simulink model "LQ_Controller"  (R2022b)
settings: Solver=ode45  StartTime=0.0  StopTime=15.0  MaxStep=0.001  RelTol=1e-5
undefined symbols (not defined in the file or in its folder): A, B, C, D, Klqi, Klqp
settings Model: Creator=emanuela  LastModifiedBy=emanuela
settings DataIOCC: SaveOutput=off  SignalLogging=off  DSMLogging=off  SaveTime=off  ReturnWorkspaceOutputs=off

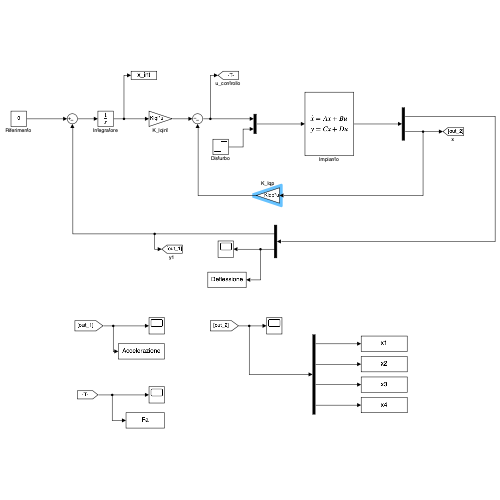
[thumbnail: Simulink's stored preview of the top-level diagram]
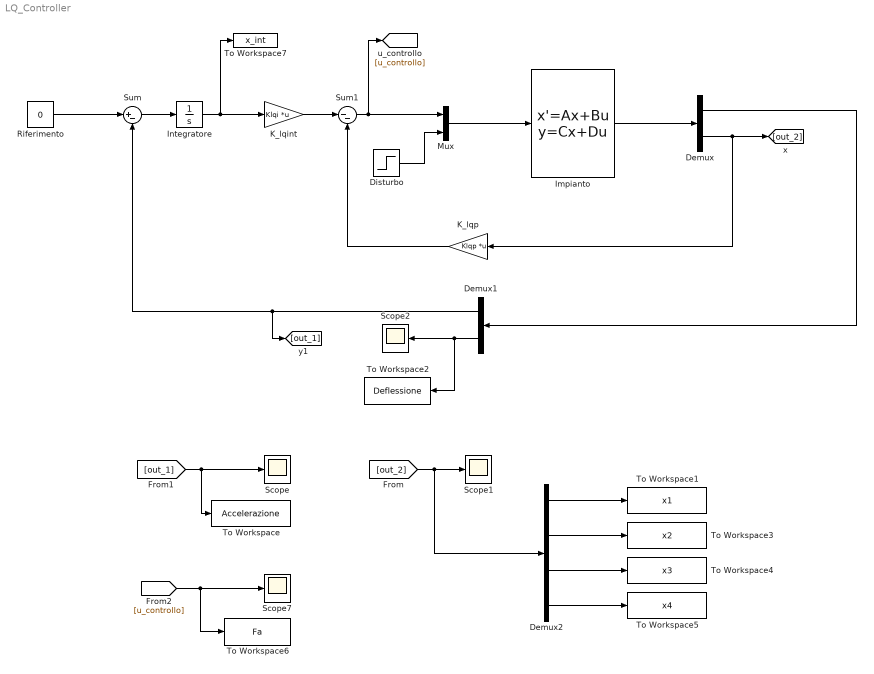
== system LQ_Controller ==
  Demux : Demux  Outputs=[2,4]
  Demux1 : Demux  Outputs=2
  Demux2 : Demux
  Disturbo : Step  Time=0  After=0.05  SampleTime=0
  Impianto : StateSpace  A=A  B=B  C=[C;eye(4)]  D=[D,;zeros(4,2)]  InitialCondition=0
  Integratore : Integrator  UpperSaturationLimit=1e6  LowerSaturationLimit=-1e6
  K_lqint : Gain  Gain=Klqi  Multiplication=Matrix(K*u)
  K_lqp : Gain  Gain=Klqp  Multiplication=Matrix(K*u)
  Mux : Mux  Inputs=2
  Riferimento : Constant  Value=0
  Scope{,1..2,7} (4 alike) : Scope
  Sum : Sum  Inputs=|+-
  Sum1 : Sum  Inputs=|--
  To Workspace : ToWorkspace  VariableName=Accelerazione  SaveFormat=Timeseries  SampleTime=-1
  To Workspace1 : ToWorkspace  VariableName=x1  SaveFormat=Timeseries  SampleTime=-1
  To Workspace2 : ToWorkspace  VariableName=Deflessione  SaveFormat=Timeseries  SampleTime=-1
  To Workspace3 : ToWorkspace  VariableName=x2  SaveFormat=Timeseries  SampleTime=-1
  To Workspace4 : ToWorkspace  VariableName=x3  SaveFormat=Timeseries  SampleTime=-1
  To Workspace5 : ToWorkspace  VariableName=x4  SaveFormat=Timeseries  SampleTime=-1
  To Workspace6 : ToWorkspace  VariableName=Fa  SaveFormat=Timeseries  SampleTime=-1
  To Workspace7 : ToWorkspace  VariableName=x_int  SaveFormat=Timeseries  SampleTime=-1
  wires:
  Demux1/2 -> To Workspace2/1, Scope2/1
  Mux/1 -> Impianto/1
  [u_controllo] -> Scope7/1, To Workspace6/1
  Impianto/1 -> Demux/1
  Demux2/1 -> To Workspace1/1
  [out_2] -> Demux2/1, Scope1/1
  Sum/1 -> Integratore/1
  Demux/1 -> Demux1/1
  Demux2/2 -> To Workspace3/1
  Demux/2 -> [out_2], K_lqp/1
  [out_1] -> To Workspace/1, Scope/1
  Demux2/4 -> To Workspace5/1
  Riferimento/1 -> Sum/1
  K_lqint/1 -> Sum1/1
  Demux2/3 -> To Workspace4/1
  K_lqp/1 -> Sum1/2
  Integratore/1 -> K_lqint/1, To Workspace7/1
  Demux1/1 -> [out_1], Sum/2
  Sum1/1 -> [u_controllo], Mux/1
  Disturbo/1 -> Mux/2
